simulink model "VCO"  (R2024a)
settings: Solver=VariableStepAuto  StartTime=0.0  StopTime=40  RelTol=1e-3
libraries: fl_lib x29, nesl_utility x25, ee_lib x14
settings Model: Creator=jacky  LastModifiedBy=jacky
settings RTWCC: GPUComputeCapability=3.5

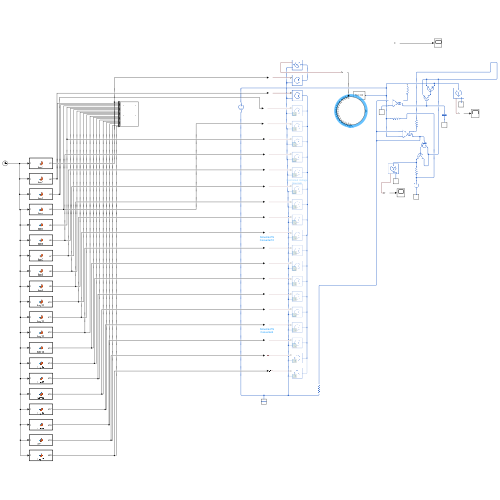
[thumbnail: Simulink's stored preview of the top-level diagram]
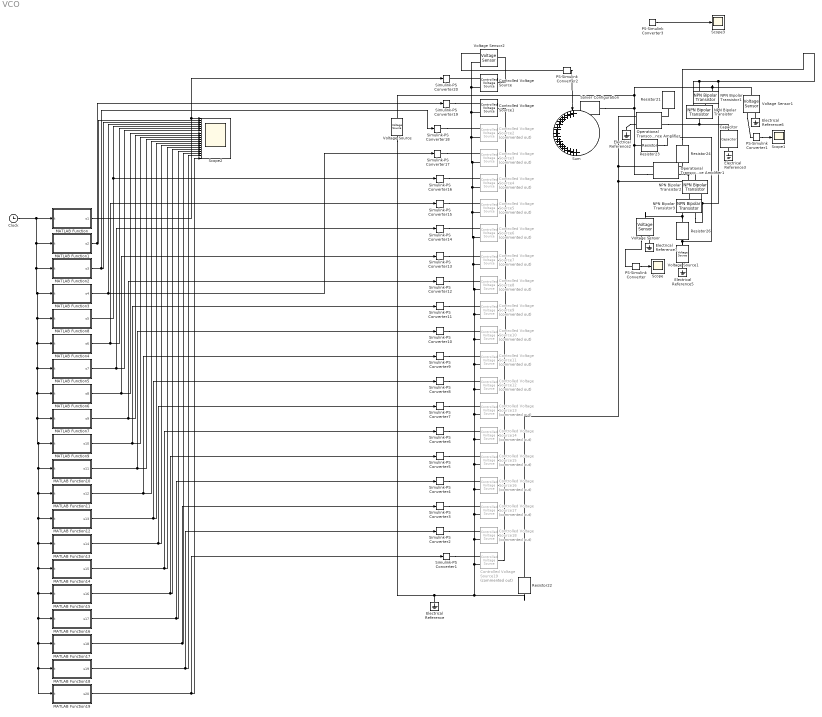
== system VCO ==
  Capacitor : ee_lib/Passive/Capacitor  cap_option=ee.enum.passive.capacitor.capOption.const  c=22 nF  Cvec=[1e-05, 1e-06] F  Vvec=[0, 10] V  CV_table_symmetry=ee.enum.passive.capacitor.tableSymmetry.yes  f_vec=[1, 10] kHz  DFext_vec=[.8, 1.2]  enable_C_tol=ee.enum.toleranceApplication.none  averaging_period=0 s  C_tol=5  tol_distribution=ee.enum.toleranceDistribution.uniform  nSigma=4  r=1e-6 Ohm  g=0 1/Ohm  maxPermissibleTemperature=85 degC  tFailOnTemperature=1 s  enable_operating_limits=ee.enum.enable.no  operating_limit_action=ee.enum.passive.reportOpLim.warn  max_working_voltage_range=[-25, 25] V  power_rating=1 W  maxTemperature=85 degC  thermalEnable=false  thermalMass=1 J/K  enable_faults=ee.enum.enable.no  fault_action=simscape.enum.assert.action.none  Cscale_faulted=100  R_faulted=1e-3 Ohm  G_faulted=0 1/Ohm  tau_fault=1e-3 s  fault_trigger=ee.enum.faults.faultTrigger.temporal  t_fault=1 s  max_permissible_voltage_range=[-100, 100] V  t_fail_on_voltage=1 s  i_specify=off  i_priority=None  i=0 A  i_nominal_specify=off  i_nominal_value=1  i_nominal_unit=A  v_specify=off  v_priority=None  v=0 V  v_nominal_specify=off  v_nominal_value=1  v_nominal_unit=V  vc_specify=off  vc_priority=High  vc=0 V  vc_nominal_specify=off  vc_nominal_value=1  vc_nominal_unit=V  T_specify=off  T_priority=None  T=298.15 K  T_nominal_specify=off  T_nominal_value=1  T_nominal_unit=K
  Clock : Clock
  Controlled Voltage Source : fl_lib/Electrical/Electrical Sources/Controlled Voltage Source
  Controlled Voltage Source1 : fl_lib/Electrical/Electrical Sources/Controlled Voltage Source
  Controlled Voltage Source{2..19} (18 alike) : fl_lib/Electrical/Electrical Sources/Controlled Voltage Source  Commented=on
  Electrical Reference{,2..3,5..7} (6 alike) : fl_lib/Electrical/Electrical Elements/Electrical Reference
  MATLAB Function : MATLAB Function  TreatAsAtomicUnit=on
  MATLAB Function1 : MATLAB Function  TreatAsAtomicUnit=on
  MATLAB Function10 : MATLAB Function  TreatAsAtomicUnit=on
  MATLAB Function11 : MATLAB Function  TreatAsAtomicUnit=on
  MATLAB Function12 : MATLAB Function  TreatAsAtomicUnit=on
  MATLAB Function13 : MATLAB Function  TreatAsAtomicUnit=on
  MATLAB Function14 : MATLAB Function  TreatAsAtomicUnit=on
  MATLAB Function15 : MATLAB Function  TreatAsAtomicUnit=on
  MATLAB Function16 : MATLAB Function  TreatAsAtomicUnit=on
  MATLAB Function17 : MATLAB Function  TreatAsAtomicUnit=on
  MATLAB Function18 : MATLAB Function  TreatAsAtomicUnit=on
  MATLAB Function19 : MATLAB Function  TreatAsAtomicUnit=on
  MATLAB Function2 : MATLAB Function  TreatAsAtomicUnit=on
  MATLAB Function3 : MATLAB Function  TreatAsAtomicUnit=on
  MATLAB Function4 : MATLAB Function  TreatAsAtomicUnit=on
  MATLAB Function5 : MATLAB Function  TreatAsAtomicUnit=on
  MATLAB Function6 : MATLAB Function  TreatAsAtomicUnit=on
  MATLAB Function7 : MATLAB Function  TreatAsAtomicUnit=on
  MATLAB Function8 : MATLAB Function  TreatAsAtomicUnit=on
  MATLAB Function9 : MATLAB Function  TreatAsAtomicUnit=on
  NPN Bipolar Transistor{,1..3} (4 alike) : ee_lib/Semiconductors & Converters/NPN Bipolar Transistor  parameterization=1  BF=100  IS=1e-14 A  VAF=200 V  hfe=100  hoe=50e-6 1/Ohm  Ic_h=1 mA  Vce_h=5 V  V1=0.55 V  I1=0.5 mA  BR=1  Tmeas=25 degC  RC=0.01 Ohm  RE=1e-4 Ohm  RB=1 Ohm  C_BC=5 pF  C_BE=5 pF  TF=0 us  TR=0 us  prmDatasheet=1  prmEquCoeff=1  hfe_T2=125  XTB=0  V1_T2=0.45 V  I1_T2=0.5 mA  Tmeas2=125 degC  EG=1.11 eV  XTI=3  TdeviceDatasheet=25 degC  TdeviceEquCoeff=25 degC  ec=1  ib_specify=off  ib_priority=None  ib=0 A  ib_nominal_specify=off  ib_nominal_value=1  ib_nominal_unit=A  ic_specify=off  ic_priority=None  ic=0 A  ic_nominal_specify=off  ic_nominal_value=1  ic_nominal_unit=A  vce_specify=off  vce_priority=None  vce=0 V  vce_nominal_specify=off  vce_nominal_value=1  vce_nominal_unit=V  vbe_specify=off  vbe_priority=None  vbe=0 V  vbe_nominal_specify=off  vbe_nominal_value=1  vbe_nominal_unit=V  Qbc_specify=off  Qbc_priority=High  Qbc=0 C  Qbc_nominal_specify=off  Qbc_nominal_value=1  Qbc_nominal_unit=uC  Qbe_specify=off  Qbe_priority=High  Qbe=0 C  Qbe_nominal_specify=off  Qbe_nominal_value=1  Qbe_nominal_unit=uC  thermal_network_parameterization=ee.enum.thermalNetworkTopology.junctionCase  Rth=[0, 10] K/W  Rth_Cauer=[1, 3, 10] K/W  Rth_Foster=[4, 6] K/W  thermal_mass_parameterization=ee.enum.thermalNetwork.timeconstant  thermal_mass=[0, 1] J/K  thermal_mass_Cauer=[.1, .3, 1] J/K  thermal_mass_Foster=[1.5, 3] J/K  thermal_time_constant=[0, 10] s  thermal_time_constant_Cauer=[1, 3, 10] s  thermal_time_constant_Foster=[6, 18] s  thermal_mass_initial_temperatures=[25, 25] degC  thermal_mass_initial_temperatures_Cauer=[25, 25, 25] degC  Tvec_initial_Foster=[25, 25, 25, 25] degC
  Operational Transconductance Amplifier : ee_lib/Integrated Circuits/Operational Transconductance Amplifier  Gm=9600 uS  Rin=25 kOhm  Rout=3 MOhm  Iabc0=500 uA  model_dynamics=ee.enum.ic.transconductanceOpampDynamics.no  f=2 MHz  slew=2 A/us  I0=0 A  Vmin=-15 V  Vmax=15 V  Ron=1 Ohm  IabcMin=0.001 uA
      settings: InternalSimscapePortConfiguration="{\"Bottom\":[],\"Left\":[{\"id\":\"p\",\"label\":\"+\",\"type\":\"foundation.electrical.electrical\"},{\"id\":\"n\",\"label\":\"-\",\"type\":\"foundation.electrical.electrical\"}],\"Right\":[{\"id\":\"Iabc\",\"label\":\"C\",\"type\":\"foundation.electrical.electrical\"},{\"id\":\"Iout\",\"label\":\"\",\"type\":\"foundation.electrical.electrical\"}],\"Top\":[]}"
  Operational Transconductance Amplifier1 : ee_lib/Integrated Circuits/Operational Transconductance Amplifier  Gm=9600 uS  Rin=25 kOhm  Rout=3 MOhm  Iabc0=500 uA  model_dynamics=ee.enum.ic.transconductanceOpampDynamics.no  f=2 MHz  slew=2 A/us  I0=0 A  Vmin=-15 V  Vmax=15 V  Ron=1 Ohm  IabcMin=0.001 uA
      settings: InternalSimscapePortConfiguration="{\"Bottom\":[],\"Left\":[{\"id\":\"p\",\"label\":\"+\",\"type\":\"foundation.electrical.electrical\"},{\"id\":\"n\",\"label\":\"-\",\"type\":\"foundation.electrical.electrical\"}],\"Right\":[{\"id\":\"Iabc\",\"label\":\"C\",\"type\":\"foundation.electrical.electrical\"},{\"id\":\"Iout\",\"label\":\"\",\"type\":\"foundation.electrical.electrical\"}],\"Top\":[]}"
  PS-Simulink Converter{,1..3} (4 alike) : nesl_utility/PS-Simulink Converter  PhysicalDomain=network_engine_domain  SubClassName=ps_output  LeftPortType=input  RightPortType=output  PseudoPeriodic=off  Frequencies=[]  VectorFormat=inherit  Unit=inherit  AffineConversion=off
  Resistor21 : ee_lib/Passive/Resistor  R=10 kOhm  enable_R_tol=ee.enum.toleranceApplication.none  R_tol=5  tol_distribution=ee.enum.toleranceDistribution.uniform  nSigma=4  enable_operating_limits=ee.enum.enable.no  operating_limit_action=ee.enum.passive.reportOpLim.warn  power_rating=1 W  max_working_voltage=100 V  enable_faults=ee.enum.enable.no  fault_action=simscape.enum.assert.action.none  R_faulted=inf Ohm  fault_trigger=ee.enum.faults.faultTrigger.temporal  t_fault=1 s  max_permissible_current=1 A  t_fail_on_current=1 s  noise_mode=ee.enum.sources.noise.Disabled  Tdevice=25 degC  sample_time=1e-3 s  repeatability=ee.enum.ic.repeatability.notRepeatable  user_seed=0  auto_seed=2915145293  faulted_specify=off  faulted_priority=None  faulted=0  power_derating_T1=70 degC  power_derating_T2=155 degC  operating_temperature_range_vec=[-50, 150] degC  alpha=3.93e-3 1/K  Tmeas=25 degC  thermal_mass=100 J/K  temperature_specify=off  temperature_priority=High  temperature=298.15 K  temperature_nominal_specify=off  temperature_nominal_value=1  temperature_nominal_unit=K
  Resistor22 : ee_lib/Passive/Resistor  R=1 kOhm  enable_R_tol=ee.enum.toleranceApplication.none  R_tol=5  tol_distribution=ee.enum.toleranceDistribution.uniform  nSigma=4  enable_operating_limits=ee.enum.enable.no  operating_limit_action=ee.enum.passive.reportOpLim.warn  power_rating=1 W  max_working_voltage=100 V  enable_faults=ee.enum.enable.no  fault_action=simscape.enum.assert.action.none  R_faulted=inf Ohm  fault_trigger=ee.enum.faults.faultTrigger.temporal  t_fault=1 s  max_permissible_current=1 A  t_fail_on_current=1 s  noise_mode=ee.enum.sources.noise.Disabled  Tdevice=25 degC  sample_time=1e-3 s  repeatability=ee.enum.ic.repeatability.notRepeatable  user_seed=0  auto_seed=4011470453  faulted_specify=off  faulted_priority=None  faulted=0  power_derating_T1=70 degC  power_derating_T2=155 degC  operating_temperature_range_vec=[-50, 150] degC  alpha=3.93e-3 1/K  Tmeas=25 degC  thermal_mass=100 J/K  temperature_specify=off  temperature_priority=High  temperature=298.15 K  temperature_nominal_specify=off  temperature_nominal_value=1  temperature_nominal_unit=K
  Resistor23 : ee_lib/Passive/Resistor  R=4700 Ohm  enable_R_tol=ee.enum.toleranceApplication.none  R_tol=5  tol_distribution=ee.enum.toleranceDistribution.uniform  nSigma=4  enable_operating_limits=ee.enum.enable.no  operating_limit_action=ee.enum.passive.reportOpLim.warn  power_rating=1 W  max_working_voltage=100 V  enable_faults=ee.enum.enable.no  fault_action=simscape.enum.assert.action.none  R_faulted=inf Ohm  fault_trigger=ee.enum.faults.faultTrigger.temporal  t_fault=1 s  max_permissible_current=1 A  t_fail_on_current=1 s  noise_mode=ee.enum.sources.noise.Disabled  Tdevice=25 degC  sample_time=1e-3 s  repeatability=ee.enum.ic.repeatability.notRepeatable  user_seed=0  auto_seed=3254469079  faulted_specify=off  faulted_priority=None  faulted=0  power_derating_T1=70 degC  power_derating_T2=155 degC  operating_temperature_range_vec=[-50, 150] degC  alpha=3.93e-3 1/K  Tmeas=25 degC  thermal_mass=100 J/K  temperature_specify=off  temperature_priority=High  temperature=298.15 K  temperature_nominal_specify=off  temperature_nominal_value=1  temperature_nominal_unit=K
  Resistor24 : ee_lib/Passive/Resistor  R=15 kOhm  enable_R_tol=ee.enum.toleranceApplication.none  R_tol=5  tol_distribution=ee.enum.toleranceDistribution.uniform  nSigma=4  enable_operating_limits=ee.enum.enable.no  operating_limit_action=ee.enum.passive.reportOpLim.warn  power_rating=1 W  max_working_voltage=100 V  enable_faults=ee.enum.enable.no  fault_action=simscape.enum.assert.action.none  R_faulted=inf Ohm  fault_trigger=ee.enum.faults.faultTrigger.temporal  t_fault=1 s  max_permissible_current=1 A  t_fail_on_current=1 s  noise_mode=ee.enum.sources.noise.Disabled  Tdevice=25 degC  sample_time=1e-3 s  repeatability=ee.enum.ic.repeatability.notRepeatable  user_seed=0  auto_seed=3191729647  faulted_specify=off  faulted_priority=None  faulted=0  power_derating_T1=70 degC  power_derating_T2=155 degC  operating_temperature_range_vec=[-50, 150] degC  alpha=3.93e-3 1/K  Tmeas=25 degC  thermal_mass=100 J/K  temperature_specify=off  temperature_priority=High  temperature=298.15 K  temperature_nominal_specify=off  temperature_nominal_value=1  temperature_nominal_unit=K
  Resistor26 : ee_lib/Passive/Resistor  R=4700 Ohm  enable_R_tol=ee.enum.toleranceApplication.none  R_tol=5  tol_distribution=ee.enum.toleranceDistribution.uniform  nSigma=4  enable_operating_limits=ee.enum.enable.no  operating_limit_action=ee.enum.passive.reportOpLim.warn  power_rating=1 W  max_working_voltage=100 V  enable_faults=ee.enum.enable.no  fault_action=simscape.enum.assert.action.none  R_faulted=inf Ohm  fault_trigger=ee.enum.faults.faultTrigger.temporal  t_fault=1 s  max_permissible_current=1 A  t_fail_on_current=1 s  noise_mode=ee.enum.sources.noise.Disabled  Tdevice=25 degC  sample_time=1e-3 s  repeatability=ee.enum.ic.repeatability.notRepeatable  user_seed=0  auto_seed=2815256101  faulted_specify=off  faulted_priority=None  faulted=0  power_derating_T1=70 degC  power_derating_T2=155 degC  operating_temperature_range_vec=[-50, 150] degC  alpha=3.93e-3 1/K  Tmeas=25 degC  thermal_mass=100 J/K  temperature_specify=off  temperature_priority=High  temperature=298.15 K  temperature_nominal_specify=off  temperature_nominal_value=1  temperature_nominal_unit=K
  Scope : Scope
  Scope1 : Scope
  Scope2 : Scope  NumInputPorts=20
  Scope3 : Scope
  Simulink-PS Converter{1..20} (20 alike) : nesl_utility/Simulink-PS Converter  PhysicalDomain=network_engine_domain  SubClassName=ps_input  LeftPortType=input  RightPortType=output  PseudoPeriodic=off  Frequencies=[]  NoiseDistribution=none  NoiseParameters=[]  Unit=1  AffineConversion=off  FilteringAndDerivatives=provide  SimscapeFilterOrder=1  InputFilterTimeConstant=0.001  UdotUserProvided=0
  Solver Configuration : nesl_utility/Solver Configuration  PhysicalDomain=network_engine_domain  SubClassName=solver  LeftPortType=input  RightPortType=generic  Tones=[]  Harmonics=[]  SimulateNoise=off  Profile=off  UseLocalSampling=off  EnableSwitchedLinearOptims=on  FrequencyDomain=off  UseCCode=off  RelTol=0.001  AbsTol=0.001  MinStep=1e-09  ToWorkspace=off  RevertToSquareIcSolve=off  NumHomotopyIterations=100  PhasorMode=off  PhasorModeNumHarmonics=1  ConsistencySolver=NEWTON_XTOL_AFTER_FTOL  IndexReductionMethod=DerivativeReplacement  DoDC=off  ResidualTolerance=1e-09  ConsistencyTolSource=GLOBAL  ConsistencyAbsTol=0.001  ConsistencyRelTol=0.001  ConsistencyTolFactor=0.001  UseLocalSolver=on  LocalSolverChoice=NE_BACKWARD_EULER_ADVANCER  ResolveIndetEquations=on  FunctionEvalNumThread=1  LocalSolverSampleTime=0.001  DoFixedCost=on  MaxNonlinIter=3  MaxModeIter=2  ComputeImpulses=off  ImpulseIterations=2  LinearAlgebra=auto  LinearAlgebraNumThread=0  EquationFormulation=NE_TIME_EF  DelaysMemoryBudget=4096  AutomaticFiltering=on  FilteringTimeConstant=0.001  PartitionStorageMethod=AS_NEEDED  PartitionMemoryBudget=1024  PartitionMethod=ROBUST  MultibodyUseLocalSolver=off  MultibodyLocalSolverChoice=ODE1  MultibodyLocalSolverSampleTime=0.001
  Sum : Sum  Inputs=|++++++++++++++++++++
  Voltage Sensor : fl_lib/Electrical/Electrical Sensors/Voltage Sensor
  Voltage Sensor1 : fl_lib/Electrical/Electrical Sensors/Voltage Sensor
  Voltage Sensor2 : fl_lib/Electrical/Electrical Sensors/Voltage Sensor
  Voltage Source : ee_lib/Sources/Voltage Source  dc_voltage=12 V  ac_voltage=0 V  ac_shift=0 rad  ac_frequency=60 Hz  noise_mode=ee.enum.sources.noise.Disabled  PSD=0 V^2/Hz  sample_time=1e-3 s  repeatability=ee.enum.sources.repeatability.NotRepeatable  user_seed=0  auto_seed=3890346746  i_specify=off  i_priority=None  i=0 A  i_nominal_specify=off  i_nominal_value=1  i_nominal_unit=A  v_specify=off  v_priority=None  v=0 V  v_nominal_specify=off  v_nominal_value=1  v_nominal_unit=V
  Voltage Source1 : ee_lib/Sources/Voltage Source  dc_voltage=-12 V  ac_voltage=0 V  ac_shift=0 rad  ac_frequency=60 Hz  noise_mode=ee.enum.sources.noise.Disabled  PSD=0 V^2/Hz  sample_time=1e-3 s  repeatability=ee.enum.sources.repeatability.NotRepeatable  user_seed=0  auto_seed=735241226  i_specify=off  i_priority=None  i=0 A  i_nominal_specify=off  i_nominal_value=1  i_nominal_unit=A  v_specify=off  v_priority=None  v=0 V  v_nominal_specify=off  v_nominal_value=1  v_nominal_unit=V
  wires:
  PS-Simulink Converter/1 -> Scope/1
  PS-Simulink Converter1/1 -> Scope1/1
  Clock/1 -> MATLAB Function19/1(t), MATLAB Function18/1(t), MATLAB Function17/1(t), MATLAB Function16/1(t), MATLAB Function15/1(t), MATLAB Function14/1(t), MATLAB Function13/1(t), MATLAB Function12/1(t), MATLAB Function11/1(t), MATLAB Function10/1(t), MATLAB Function9/1(t), MATLAB Function7/1(t), MATLAB Function6/1(t), MATLAB Function5/1(t), MATLAB Function4/1(t), MATLAB Function8/1(t), MATLAB Function3/1(t), MATLAB Function2/1(t), MATLAB Function1/1(t), MATLAB Function/1(t)
  MATLAB Function/1(s1) -> Simulink-PS Converter20/1, Scope2/1
  MATLAB Function1/1(s2) -> Simulink-PS Converter19/1, Scope2/2
  MATLAB Function2/1(s3) -> Simulink-PS Converter18/1, Scope2/3
  MATLAB Function8/1(s5) -> Simulink-PS Converter16/1, Scope2/5
  MATLAB Function4/1(s6) -> Simulink-PS Converter15/1, Scope2/6
  MATLAB Function5/1(s7) -> Simulink-PS Converter14/1, Scope2/7
  MATLAB Function7/1(s9) -> Simulink-PS Converter12/1, Scope2/9
  MATLAB Function9/1(s10) -> Simulink-PS Converter11/1, Scope2/10
  MATLAB Function10/1(s11) -> Simulink-PS Converter10/1, Scope2/11
  MATLAB Function11/1(s12) -> Simulink-PS Converter9/1, Scope2/12
  MATLAB Function12/1(s13) -> Simulink-PS Converter8/1, Scope2/13
  MATLAB Function13/1(s14) -> Simulink-PS Converter7/1, Scope2/14
  MATLAB Function14/1(s15) -> Simulink-PS Converter6/1, Scope2/15
  MATLAB Function15/1(s16) -> Simulink-PS Converter5/1, Scope2/16
  MATLAB Function16/1(s17) -> Simulink-PS Converter4/1, Scope2/17
  MATLAB Function17/1(s18) -> Simulink-PS Converter3/1, Scope2/18
  MATLAB Function18/1(s19) -> Simulink-PS Converter2/1, Scope2/19
  MATLAB Function19/1(s20) -> Simulink-PS Converter1/1, Scope2/20
  MATLAB Function3/1(s4) -> Simulink-PS Converter17/1, Scope2/4
  MATLAB Function6/1(s8) -> Simulink-PS Converter13/1, Scope2/8
  PS-Simulink Converter3/1 -> Scope3/1
  PS-Simulink Converter2/1 -> Sum/1
  connections:
  Controlled Voltage Source1/LConn1 -- Controlled Voltage Source19/LConn1 -- Controlled Voltage Source18/LConn1 -- Controlled Voltage Source17/LConn1 -- Controlled Voltage Source16/LConn1 -- Controlled Voltage Source15/LConn1 -- Controlled Voltage Source14/LConn1 -- Controlled Voltage Source13/LConn1 -- Controlled Voltage Source12/LConn1 -- Controlled Voltage Source11/LConn1 -- Controlled Voltage Source10/LConn1 -- Controlled Voltage Source9/LConn1 -- Controlled Voltage Source8/LConn1 -- Controlled Voltage Source7/LConn1 -- Controlled Voltage Source6/LConn1 -- Controlled Voltage Source5/LConn1 -- Controlled Voltage Source4/LConn1 -- Controlled Voltage Source3/LConn1 -- Controlled Voltage Source2/LConn1
  Resistor24/LConn1 -- NPN Bipolar Transistor/RConn1 -- NPN Bipolar Transistor1/RConn1 -- NPN Bipolar Transistor3/RConn1 -- NPN Bipolar Transistor2/RConn1
  Operational Transconductance Amplifier1/LConn1 -- Operational Transconductance Amplifier1/RConn2 -- NPN Bipolar Transistor2/LConn1 -- Resistor22/LConn1 -- Operational Transconductance Amplifier/LConn1
  Operational Transconductance Amplifier/LConn2 -- Electrical Reference2/LConn1
  Operational Transconductance Amplifier/RConn1 -- Resistor21/RConn1
  Capacitor/LConn1 -- Operational Transconductance Amplifier/RConn2 -- NPN Bipolar Transistor/LConn1
  NPN Bipolar Transistor/RConn2 -- NPN Bipolar Transistor1/LConn1
  Electrical Reference3/LConn1 -- Capacitor/RConn1
  Resistor24/RConn1 -- Operational Transconductance Amplifier1/RConn1
  NPN Bipolar Transistor2/RConn2 -- NPN Bipolar Transistor3/LConn1
  Operational Transconductance Amplifier1/LConn2 -- Solver Configuration/RConn1 -- Voltage Sensor1/LConn1 -- NPN Bipolar Transistor1/RConn2 -- Voltage Source/LConn1 -- Resistor23/LConn1
  NPN Bipolar Transistor3/RConn2 -- Voltage Sensor/LConn1 -- Resistor26/LConn1
  Resistor26/RConn1 -- Resistor23/RConn1 -- Voltage Source1/LConn1
  Electrical Reference6/LConn1 -- Voltage Sensor1/RConn2
  Electrical Reference7/LConn1 -- Voltage Sensor/RConn2
  Voltage Sensor/RConn1 -- PS-Simulink Converter/LConn1
  Voltage Sensor1/RConn1 -- PS-Simulink Converter1/LConn1
  Voltage Source1/RConn1 -- Electrical Reference5/LConn1
  Controlled Voltage Source/RConn1 -- Simulink-PS Converter20/RConn1
  Voltage Sensor2/RConn1 -- PS-Simulink Converter2/LConn1
  Controlled Voltage Source/RConn2 -- Voltage Sensor2/RConn2 -- Controlled Voltage Source1/RConn2 -- Resistor22/RConn1 -- Voltage Source/RConn1 -- Electrical Reference/LConn1 -- Controlled Voltage Source19/RConn2 -- Controlled Voltage Source18/RConn2 -- Controlled Voltage Source17/RConn2 -- Controlled Voltage Source16/RConn2 -- Controlled Voltage Source15/RConn2 -- Controlled Voltage Source14/RConn2 -- Controlled Voltage Source13/RConn2 -- Controlled Voltage Source12/RConn2 -- Controlled Voltage Source11/RConn2 -- Controlled Voltage Source10/RConn2 -- Controlled Voltage Source9/RConn2 -- Controlled Voltage Source8/RConn2 -- Controlled Voltage Source7/RConn2 -- Controlled Voltage Source6/RConn2 -- Controlled Voltage Source5/RConn2 -- Controlled Voltage Source4/RConn2 -- Controlled Voltage Source3/RConn2 -- Controlled Voltage Source2/RConn2
  Simulink-PS Converter19/RConn1 -- Controlled Voltage Source1/RConn1
  Simulink-PS Converter1/RConn1 -- Controlled Voltage Source19/RConn1
  Simulink-PS Converter14/RConn1 -- Controlled Voltage Source6/RConn1
  Simulink-PS Converter15/RConn1 -- Controlled Voltage Source5/RConn1
  Simulink-PS Converter16/RConn1 -- Controlled Voltage Source4/RConn1
  Simulink-PS Converter17/RConn1 -- Controlled Voltage Source3/RConn1
  Simulink-PS Converter18/RConn1 -- Controlled Voltage Source2/RConn1
  Simulink-PS Converter13/RConn1 -- Controlled Voltage Source7/RConn1
  Simulink-PS Converter12/RConn1 -- Controlled Voltage Source8/RConn1
  Simulink-PS Converter11/RConn1 -- Controlled Voltage Source9/RConn1
  Simulink-PS Converter10/RConn1 -- Controlled Voltage Source10/RConn1
  Simulink-PS Converter9/RConn1 -- Controlled Voltage Source11/RConn1
  Simulink-PS Converter8/RConn1 -- Controlled Voltage Source12/RConn1
  Simulink-PS Converter7/RConn1 -- Controlled Voltage Source13/RConn1
  Simulink-PS Converter6/RConn1 -- Controlled Voltage Source14/RConn1
  Simulink-PS Converter5/RConn1 -- Controlled Voltage Source15/RConn1
  Simulink-PS Converter2/RConn1 -- Controlled Voltage Source18/RConn1
  Simulink-PS Converter3/RConn1 -- Controlled Voltage Source17/RConn1
  Simulink-PS Converter4/RConn1 -- Controlled Voltage Source16/RConn1
  Controlled Voltage Source/LConn1 -- Voltage Sensor2/LConn1

== matlab function VCO/MATLAB Function11 ==
  data: t input; s12 output
function s12 = key12(t)

if 22<t && t<23
    s12 = 5.4
else
    s12 = 0
end

== matlab function VCO/MATLAB Function12 ==
  data: t input; s13 output
function s13 = key13(t)

if 24<t && t<25
    s13 = 4.8
else
    s13 = 0
end

== matlab function VCO/MATLAB Function13 ==
  data: t input; s14 output
function s14 = key14(t)

if 26<t && t<27
    s14 = 4.2
else
    s14 = 0
end

== matlab function VCO/MATLAB Function14 ==
  data: t input; s15 output
function s15 = key15(t)

if 28<t && t<29
    s15 = 3.6
else
    s15 = 0
end

== matlab function VCO/MATLAB Function15 ==
  data: t input; s16 output
function s16 = key16(t)

if 30<t && t<31
    s16 = 3
else
    s16 = 0
end

== matlab function VCO/MATLAB Function16 ==
  data: t input; s17 output
function s17 = key17(t)

if 32<t && t<33
    s17 = 2.4
else
    s17 = 0
end

== matlab function VCO/MATLAB Function17 ==
  data: t input; s18 output
function s18 = key18(t)

if 34<t && t<35
    s18 = 1.8
else
    s18 = 0
end

== matlab function VCO/MATLAB Function18 ==
  data: t input; s19 output
function s19 = key19(t)

if 36<t && t<37
    s19 = 1.2
else
    s19 = 0
end

== matlab function VCO/MATLAB Function19 ==
  data: t input; s20 output
function s20 = key20(t)

if 38<t && t<39
    s20 = 0.6
else
    s20 = 0
end

== matlab function VCO/MATLAB Function1 ==
  data: t input; s2 output
function s2= key2(t)

if 3>t && t>2
    s2 = 11.4
else 
    s2 = 0
end

== matlab function VCO/MATLAB Function ==
  data: t input; s1 output
function s1= key1(t)

if t<1
    s1 = 12
else
    s1 = 0
end

%{
if u == 1
    keys = [0,1,0,0,0,0,0,0,0,0,0,0,0,0,0,0,0,0,0,0]
end
if u == 1
    keys = [0,0,1,0,0,0,0,0,0,0,0,0,0,0,0,0,0,0,0,0]
end
if u == 1
    keys = [0,0,0,1,0,0,0,0,0,0,0,0,0,0,0,0,0,0,0,0]
end
if u == 1
    keys = [0,0,0,0,1,0,0,0,0,0,0,0,0,0,0,0,0,0,0,0]
end
if u == 1
    keys = [0,0,0,0,0,1,0,0,0,0,0,0,0,0,0,0,0,0,0,0]
end
if u == 1
    keys = [0,0,0,0,0,0,1,0,0,0,0,0,0,0,0,0,0,0,0,0]
end
if u == 1
    keys = [0,0,0,0,0,0,0,1,0,0,0,0,0,0,0,0,0,0,0,0]
end
if u == 1
    keys = [0,0,0,0,0,0,0,0,1,0,0,0,0,0,0,0,0,0,0,0]
end
if u == 1
    keys = [0,0,0,0,0,0,0,0,0,1,0,0,0,0,0,0,0,0,0,0]
end
if u == 1
    keys = [0,0,0,0,0,0,0,0,0,0,1,0,0,0,0,0,0,0,0,0]
end
if u == 1
    keys = [0,0,0,0,0,0,0,0,0,0,0,1,0,0,0,0,0,0,0,0]
end
if u == 1
    keys = [0,0,0,0,0,0,0,0,0,0,0,0,1,0,0,0,0,0,0,0]
end
if u == 1
    keys = [0,0,0,0,0,0,0,0,0,0,0,0,0,1,0,0,0,0,0,0]
end
if u == 1
    keys = [0,0,0,0,0,0,0,0,0,0,0,0,0,0,1,0,0,0,0,0]
end
if u == 1
    keys = [0,0,0,0,0,0,0,0,0,0,0,0,0,0,0,1,0,0,0,0]
end
if u == 1
    keys = [0,0,0,0,0,0,0,0,0,0,0,0,0,0,0,0,1,0,0,0]
end
if u == 1
    keys = [0,0,0,0,0,0,0,0,0,0,0,0,0,0,0,0,0,1,0,0]
end
if u == 1
    keys = [0,0,0,0,0,0,0,0,0,0,0,0,0,0,0,0,0,0,1,0]
end
if u == 1
    keys = [0,0,0,0,0,0,0,0,0,0,0,0,0,0,0,0,0,0,0,1]
end
%}

== matlab function VCO/MATLAB Function2 ==
  data: t input; s3 output
function s3= key3(t)

if 4<t && t<5
    s3 = 10.8
else
    s3 = 0
end

== matlab function VCO/MATLAB Function3 ==
  data: t input; s4 output
function s4= key4(t)

if 6<t && t<7
    s4 = 10.2
else
    s4 = 0
end

== matlab function VCO/MATLAB Function4 ==
  data: t input; s6 output
function s6= key6(t)

if 10<t && t<11
    s6 = 9
else
    s6 = 0
end

== matlab function VCO/MATLAB Function5 ==
  data: t input; s7 output
function s7= key7(t)

if 12<t && t<13
    s7 = 8.4
else
    s7 = 0
end

== matlab function VCO/MATLAB Function6 ==
  data: t input; s8 output
function s8 = key8(t)

if 14<t && t<15
    s8 = 7.8
else
    s8 = 0
end

== matlab function VCO/MATLAB Function7 ==
  data: t input; s9 output
function s9 = key9(t)

if 16<t && t<17
    s9 = 7.2
else
    s9 = 0
end

== matlab function VCO/MATLAB Function8 ==
  data: t input; s5 output
function s5= key5(t)

if 8<t && t<9
    s5 = 9.6
else
    s5 = 0
end

== matlab function VCO/MATLAB Function9 ==
  data: t input; s10 output
function s10 = key10(t)

if 18<t && t<19
    s10 = 6.6
else
    s10 = 0
end

== matlab function VCO/MATLAB Function10 ==
  data: t input; s11 output
function s11 = key11(t)

if 20<t && t<21
    s11 = 6
else
    s11 = 0
end
